simulink model "debug_IMUCalib_legacy"  (Simulink 8.3)
settings: Solver=FixedStepDiscrete  StartTime=0.0  StopTime=inf  FixedStep=0.01  RelTol=1e-3
InitFcn:
  | ROBOT_DOF=23;
libraries: WBToolboxLibrary x2
settings Model: Creator=DanielePucci  LastModifiedBy=gnava  CovSFcnEnable=on
settings DataIOCC: SaveFormat=StructureWithTime  SignalLoggingSaveFormat=Dataset
settings DebuggingCC: UnderspecifiedInitializationDetection=Simplified  MergeDetectMultiDrivingBlocksExec=error  SolverPrmCheckMsg=none  FrameProcessingCompatibilityMsg=error  StateNameClashWarn=none
settings HardwareCC: ProdBitPerPointer=64  ProdLargestAtomicFloat=Float  ProdIntDivRoundTo=Zero  ProdEndianess=LittleEndian  ProdHWDeviceType=Specified
settings GRTTargetCC: GeneratePreprocessorConditionals=Use local settings  CombineOutputUpdateFcns=on  GRTInterface=off

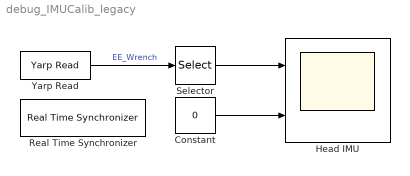
== system debug_IMUCalib_legacy ==
  Constant : Constant  Value=0
  Head IMU : Scope  NumInputPorts=2
      settings: TimeRange=auto  ShowLegends=on  MaxDataPoints=5000  SaveToWorkspace=off  YMin=-0.27073~-5  YMax=0.28409~5  SampleTime=-1
  Real Time Synchronizer : WBToolboxLibrary/Utilities/Real Time Synchronizer  period=0.01
  Selector : Selector  InputPortWidth=12  IndexOptions=Index vector (dialog)  Indices=[4:6]  OutputSizes=1
  Yarp Read : WBToolboxLibrary/Utilities/Yarp Read  portName='/icub/inertial'  signalSize=12  blocking=off  timestamp=off  autoconnect=on  errorOnConnection=off
  wires:
  Yarp Read/1 -> Selector/1  "EE_Wrench"
  Selector/1 -> Head IMU/1
  Constant/1 -> Head IMU/2
